simulink model "capitol2prob4"  (R2013a)
settings: Solver=ode45  StartTime=0.0  StopTime=200  RelTol=1e-3
undefined symbols (not defined in the file): des, gcbh
settings Model: Creator=user  LastModifiedBy=user

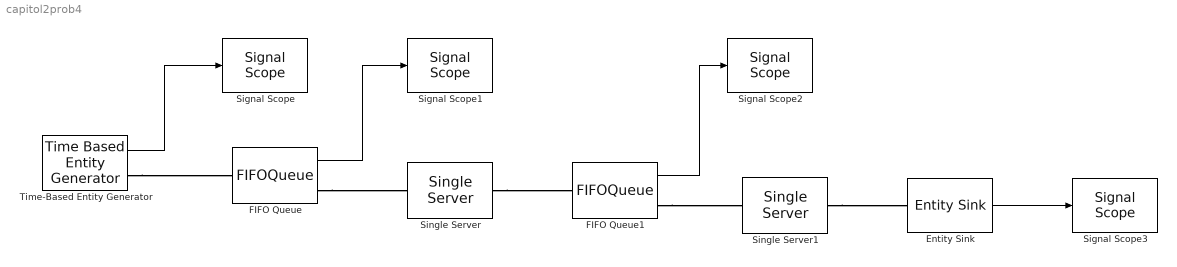
== system capitol2prob4 ==
  Entity Sink : EntitySink  StatNumberArrived=on
  FIFO Queue : FIFOQueue  StatNumberInBlock=on
      settings: OutputPortMap=o1
  FIFO Queue1 : FIFOQueue  StatNumberInBlock=on
      settings: OutputPortMap=o1
  Signal Scope{,1..3} (4 alike) : SignalScope  LoadFcn=des.scope.CallbackSupport('seLoadFcn',gcbh)  StartFcn=des.scope.CallbackSupport('seStartFcn',gcbh)  StopFcn=des.scope.CallbackSupport('seStopFcn',gcbh)
      settings: CopyFcn=des.scope.CallbackSupport('seCopyFcn',gcbh)  DeleteFcn=des.scope.CallbackSupport('seDeleteFcn',gcbh)  PreSaveFcn=des.scope.CallbackSupport('sePreSaveFcn',gcbh)  NameChangeFcn=des.scope.CallbackSupport('seNameChangeFcn',gcbh)  OpenFcn=des.scope.CallbackSupport('seOpenFcn',gcbh)
  Single Server : SingleServer  ServiceTime=17
  Single Server1 : SingleServer  ServiceTime=15
  Time-Based Entity Generator : TimeBasedEntityGenerator  Distribution=Uniform  Minimum=12  Maximum=22  StatNumberDeparted=on
  wires:
  Time-Based Entity Generator/1 -> Signal Scope/1
  FIFO Queue/1 -> Signal Scope1/1
  FIFO Queue1/1 -> Signal Scope2/1
  Entity Sink/1 -> Signal Scope3/1
  connections:
  Time-Based Entity Generator/RConn1 -- FIFO Queue/LConn1
  FIFO Queue/RConn1 -- Single Server/LConn1
  Single Server/RConn1 -- FIFO Queue1/LConn1
  FIFO Queue1/RConn1 -- Single Server1/LConn1
  Single Server1/RConn1 -- Entity Sink/LConn1
